simulink model "barrel_switcher_xblock_models"  (Simulink 7.4)
settings: Solver=ode45  StartTime=0.0  StopTime=10.0  RelTol=1e-3
libraries: xbsIndex_r4 x35
settings Model: Creator=chenhong  LastModifiedBy=chenhong

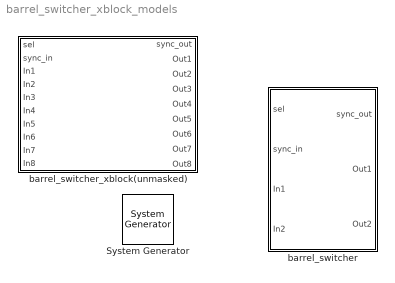
== system barrel_switcher_xblock_models ==
  " System Generator" : xbsIndex_r4/ System Generator  Tag=genX  SystemSampleTime=-1  xilinxfamily=Virtex6  part=xc6vsx315t  speed=-3  package=ff1156  synthesis_tool=XST  clock_wrapper=Clock Enables  directory=./netlist  testbench=off  simulink_period=1  sysclk_period=10  dcm_input_clock_period=10  incr_netlist=off  trim_vbits=Everywhere in SubSystem  dbl_ovrd=According to Block Masks  core_generation=According to Block Masks  run_coregen=off  deprecated_control=off  eval_field=0  block_type=sysgen
      settings: block_version=11.4
  barrel_switcher : Subsystem  mask(barrel_switcher){n_inputs=1}
      mask prompts: n_inputs "Number of Inputs: (2^?)"
      mask help:
      | Shifts input to right by amount specified on sel,
      | wrapping around into higher order bits.
      mask init:
      | config.source=str2func('barrel_switcher_init_xblock');
      | config.toplevel=gcb;
      | xBlock(config, ...
      |     {n_inputs});
      settings: AttributesFormatString=n_inputs=2
      mask Help: eval('xlWeb(''http://casper.berkeley.edu/wiki/Barrel_switcher'')')
  barrel_switcher_xblock(unmasked) : Subsystem

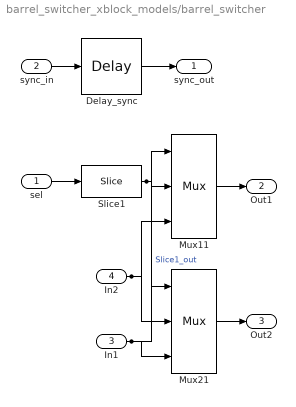
== system barrel_switcher_xblock_models/barrel_switcher ==
  sel : Inport  OutDataType=sfix(16)  OutScaling=2^0
  sync_in : Inport  Port=2  OutDataType=sfix(16)  OutScaling=2^0
  In1 : Inport  Port=3  OutDataType=sfix(16)  OutScaling=2^0
  In2 : Inport  Port=4  OutDataType=sfix(16)  OutScaling=2^0
  Delay_sync : xbsIndex_r4/Delay  en=off  latency=1  dbl_ovrd=off  reg_retiming=off  block_type=delay
      settings: block_version=11.4
  Mux11 : xbsIndex_r4/Mux  inputs=2  en=off  latency=1  precision=Full  arith_type="Signed  (2's comp)"  n_bits=8  bin_pt=2  quantization=Truncate  overflow=Wrap  dbl_ovrd=off  block_type=mux
      settings: block_version=11.4
  Mux21 : xbsIndex_r4/Mux  inputs=2  en=off  latency=1  precision=Full  arith_type="Signed  (2's comp)"  n_bits=8  bin_pt=2  quantization=Truncate  overflow=Wrap  dbl_ovrd=off  block_type=mux
      settings: block_version=11.4
  Slice1 : xbsIndex_r4/Slice  nbits=1  boolean_output=off  mode=Upper Bit Location + Width  bit1=-0  base1=MSB of Input  bit0=0  base0=LSB of Input  dbl_ovrd=off  block_type=slice
  sync_out : Outport  OutDataType=sfix(16)  OutScaling=2^0
  Out1 : Outport  Port=2  OutDataType=sfix(16)  OutScaling=2^0
  Out2 : Outport  Port=3  OutDataType=sfix(16)  OutScaling=2^0
  wires:
  Slice1/1 -> Mux21/1, Mux11/1  "Slice1_out"
  In1/1 -> Mux21/3, Mux11/2
  In2/1 -> Mux21/2, Mux11/3
  Mux21/1 -> Out2/1
  Mux11/1 -> Out1/1
  sel/1 -> Slice1/1
  Delay_sync/1 -> sync_out/1
  sync_in/1 -> Delay_sync/1

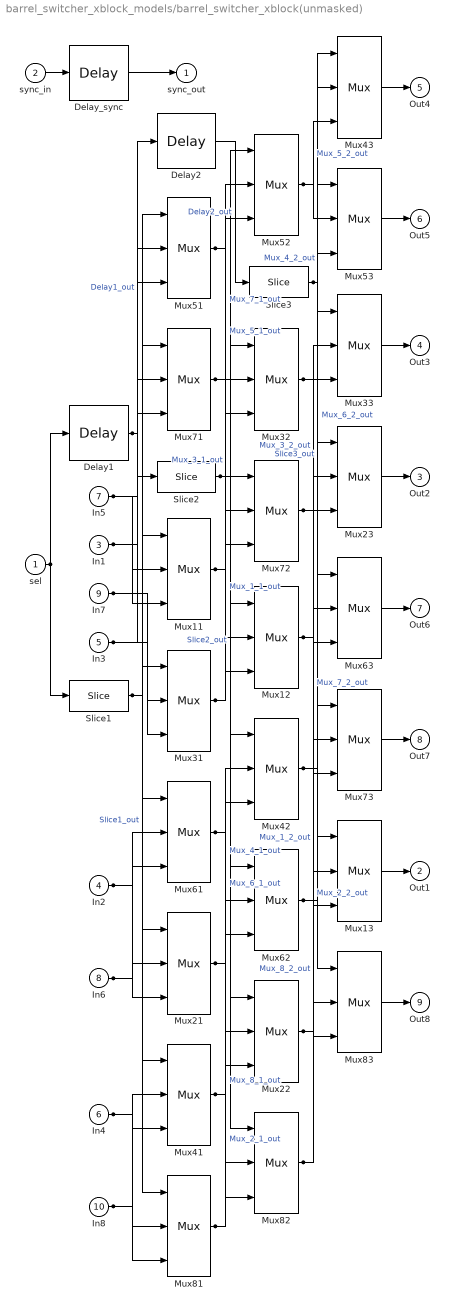
== system barrel_switcher_xblock_models/barrel_switcher_xblock(unmasked) ==
  sel : Inport
  sync_in : Inport  Port=2
  In1 : Inport  Port=3
  In2 : Inport  Port=4
  In3 : Inport  Port=5
  In4 : Inport  Port=6
  In5 : Inport  Port=7
  In6 : Inport  Port=8
  In7 : Inport  Port=9
  In8 : Inport  Port=10
  Delay1 : xbsIndex_r4/Delay  en=off  latency=1  dbl_ovrd=off  reg_retiming=off  block_type=delay
      settings: block_version=11.4
  Delay2 : xbsIndex_r4/Delay  en=off  latency=1  dbl_ovrd=off  reg_retiming=off  block_type=delay
      settings: block_version=11.4
  Delay_sync : xbsIndex_r4/Delay  en=off  latency=1  dbl_ovrd=off  reg_retiming=off  block_type=delay
      settings: block_version=11.4
  Mux{11..13,21..23,31..33,41..43,51..53,61..63,71..73,81..83} (24 alike) : xbsIndex_r4/Mux  inputs=2  en=off  latency=1  precision=Full  arith_type="Signed  (2's comp)"  n_bits=8  bin_pt=2  quantization=Truncate  overflow=Wrap  dbl_ovrd=off  block_type=mux
      settings: block_version=11.4
  Slice1 : xbsIndex_r4/Slice  nbits=1  boolean_output=off  mode=Upper Bit Location + Width  bit1=-0  base1=MSB of Input  bit0=0  base0=LSB of Input  dbl_ovrd=off  block_type=slice
  Slice2 : xbsIndex_r4/Slice  nbits=1  boolean_output=off  mode=Upper Bit Location + Width  bit1=-1  base1=MSB of Input  bit0=0  base0=LSB of Input  dbl_ovrd=off  block_type=slice
  Slice3 : xbsIndex_r4/Slice  nbits=1  boolean_output=off  mode=Upper Bit Location + Width  bit1=-2  base1=MSB of Input  bit0=0  base0=LSB of Input  dbl_ovrd=off  block_type=slice
  sync_out : Outport
  Out1 : Outport  Port=2
  Out2 : Outport  Port=3
  Out3 : Outport  Port=4
  Out4 : Outport  Port=5
  Out5 : Outport  Port=6
  Out6 : Outport  Port=7
  Out7 : Outport  Port=8
  Out8 : Outport  Port=9
  wires:
  sel/1 -> Delay1/1, Slice1/1
  Delay1/1 -> Delay2/1, Slice2/1  "Delay1_out"
  Slice1/1 -> Mux81/1, Mux71/1, Mux51/1, Mux31/1, Mux21/1, Mux11/1, Mux41/1, Mux61/1  "Slice1_out"
  Slice2/1 -> Mux62/1, Mux42/1, Mux22/1, Mux12/1, Mux32/1, Mux52/1, Mux72/1, Mux82/1  "Slice2_out"
  Slice3/1 -> Mux83/1, Mux73/1, Mux63/1, Mux43/1, Mux23/1, Mux13/1, Mux33/1, Mux53/1  "Slice3_out"
  Mux22/1 -> Mux13/3, Mux23/2  "Mux_2_2_out"
  Mux31/1 -> Mux32/2, Mux12/3  "Mux_3_1_out"
  Mux32/1 -> Mux33/2, Mux23/3  "Mux_3_2_out"
  Mux41/1 -> Mux22/3, Mux42/2  "Mux_4_1_out"
  Mux42/1 -> Mux33/3, Mux43/2  "Mux_4_2_out"
  In5/1 -> Mux11/3, Mux51/2
  In1/1 -> Mux51/3, Mux11/2
  Mux51/1 -> Mux52/2, Mux32/3  "Mux_5_1_out"
  Mux52/1 -> Mux53/2, Mux43/3  "Mux_5_2_out"
  In6/1 -> Mux61/2, Mux21/3
  In2/1 -> Mux21/2, Mux61/3
  Mux61/1 -> Mux42/3, Mux62/2  "Mux_6_1_out"
  Mux62/1 -> Mux53/3, Mux63/2  "Mux_6_2_out"
  In7/1 -> Mux31/3, Mux71/2
  In3/1 -> Mux71/3, Mux31/2
  Mux71/1 -> Mux72/2, Mux52/3  "Mux_7_1_out"
  Mux11/1 -> Mux12/2, Mux72/3  "Mux_1_1_out"
  Mux72/1 -> Mux63/3, Mux73/2  "Mux_7_2_out"
  In8/1 -> Mux41/3, Mux81/2
  In4/1 -> Mux81/3, Mux41/2
  Mux81/1 -> Mux82/2, Mux62/3  "Mux_8_1_out"
  Mux21/1 -> Mux22/2, Mux82/3  "Mux_2_1_out"
  Mux82/1 -> Mux73/3, Mux83/2  "Mux_8_2_out"
  Mux12/1 -> Mux83/3, Mux13/2  "Mux_1_2_out"
  Mux73/1 -> Out7/1
  Mux63/1 -> Out6/1
  Mux43/1 -> Out4/1
  Mux23/1 -> Out2/1
  Mux13/1 -> Out1/1
  sync_in/1 -> Delay_sync/1
  Delay_sync/1 -> sync_out/1
  Delay2/1 -> Slice3/1  "Delay2_out"
  Mux33/1 -> Out3/1
  Mux53/1 -> Out5/1
  Mux83/1 -> Out8/1
